simulink model "Furnace"  (R2020a)
settings: Solver=ode15s  StartTime=0  StopTime=27000  FixedStep=0.1  MaxStep=20  MinStep=1e-13  RelTol=1e-08  AbsTol=1e-09
undefined symbols (not defined in the file): agnostic_lqe_params, cont_reg, disturbance_type, F_aI_pid, F_aII_pid, input_type, k, lqe_params, LQR_params, LQRAgnostic_params, MPC_type, MPCDiscrete_function_parameters, MPCDiscreteAgnostic_function_parameters, MPCDiscreteDiffIntegralAgnostic_function_parameters, original_LQR_params, output_type, reg, single_butter_ss
libraries: simulink x35, cstblocks x10, mpclib x3
(part 3 of 8)

== system Furnace/Plant2/Turbine ==
  T_SH : Inport
  F_SH : Inport  Port=2
  p_drum : Inport  Port=3
  Scope : Scope
  Sum : Sum
  Transport Delay1 : TransportDelay  DelayTime=3  BufferSize=2048
  Transport Delay2 : TransportDelay  DelayTime=3  BufferSize=2048
  Turbine : MATLAB Function  TreatAsAtomicUnit=on
  W_net : Scope
  eta_TURB : Constant  Value=k.eta_TURB
  p_HP : Constant  Value=k.p_HP
  p_LP : Constant  Value=k.p_LP
  F_turb : Outport  VectorParamsAs1DForOutWhenUnconnected=off
  wires:
  T_SH/1 -> Turbine/1(T_SH)
  Turbine/1(W_el) -> Transport Delay1/1
  p_drum/1 -> Turbine/3(p_drum)
  F_SH/1 -> Transport Delay2/1, Turbine/2(F_SH)
  p_LP/1 -> Turbine/5(p_LP)
  Transport Delay1/1 -> Sum/1
  Transport Delay2/1 -> F_turb/1
  p_HP/1 -> Turbine/4(p_HP)
  Turbine/2(Q_turb) -> Scope/1
  eta_TURB/1 -> Turbine/6(eta_TURB)
  [W_fan] -> Sum/2
  Sum/1 -> W_net/1

== system Furnace/Actuator dynamics/Secondary air/Flue gas fan ==
  note: rpm of impeller
  note: Shaft torque
  PID signal : Inport
  Alpha : Gain  Gain=k.alpha_est_aII.*100
  Constant : Constant  Value=k.omega_T_aII
  Divide : Product  Inputs=*/
  Efficiency : Gain  Gain=k.mu_eff
  Gain : Gain  Gain=1/(k.I_aII)
  Gain4 : Gain  Gain=60/(2*pi)
  Integrator : Integrator  InitialCondition=reg.F_aII_fan_model_int
  "Linear mapping from rpm to volume flow " : Gain  Gain=k.map_aII
  "Maksimum power " : Gain  Gain=k.Pmax_aII
  Plus2 : Sum  Inputs=+-
  Square : Math  Operator=square  SignedPower=on  SaturateOnIntegerOverflow=on
  Square1 : Math  Operator=square  SignedPower=on  SaturateOnIntegerOverflow=on
  Static pressure converter : Gain  Gain=k.alpha_est_aII*2*3.1415/k.map_aII
  Switch : Switch  Criteria=u2 > Threshold  Threshold=k.omega_T_aII
  Volume flow : Outport  VectorParamsAs1DForOutWhenUnconnected=off
  Pressure difference : Outport  Port=2  VectorParamsAs1DForOutWhenUnconnected=off
  Power consumption : Outport  Port=3  VectorParamsAs1DForOutWhenUnconnected=off
  wires:
  Integrator/1 -> Square/1, Gain4/1, Switch/2, Switch/1, Square1/1
  Divide/1 -> Plus2/1
  Gain4/1 -> "Linear mapping from rpm to volume flow "/1
  Square/1 -> Static pressure converter/1
  Efficiency/1 -> Pressure difference/1
  "Maksimum power "/1 -> Power consumption/1, Divide/1
  Static pressure converter/1 -> Efficiency/1
  Alpha/1 -> Plus2/2
  Square1/1 -> Alpha/1
  Gain/1 -> Integrator/1
  Plus2/1 -> Gain/1
  PID signal/1 -> "Maksimum power "/1
  "Linear mapping from rpm to volume flow "/1 -> Volume flow/1
  Switch/1 -> Divide/2
  Constant/1 -> Switch/3

== system Furnace/Actuator dynamics/Waste and Primary air/Flue gas fan ==
  note: rpm of impeller
  note: Shaft torque
  PID signal : Inport
  Alpha : Gain  Gain=k.alpha_est_aII.*100
  Constant : Constant  Value=k.omega_T_aII
  Divide : Product  Inputs=*/
  Efficiency : Gain  Gain=k.mu_eff
  Gain : Gain  Gain=1/(k.I_aII)
  Gain4 : Gain  Gain=60/(2*pi)
  Integrator : Integrator  InitialCondition=reg.F_aI_fan_model_int
  "Linear mapping from rpm to volume flow " : Gain  Gain=k.map_aII
  "Maksimum power " : Gain  Gain=k.Pmax_aII
  Plus2 : Sum  Inputs=+-
  Square : Math  Operator=square  SignedPower=on  SaturateOnIntegerOverflow=on
  Square1 : Math  Operator=square  SignedPower=on  SaturateOnIntegerOverflow=on
  Static pressure converter : Gain  Gain=k.alpha_est_aII*2*3.1415/k.map_aII
  Switch : Switch  Criteria=u2 > Threshold  Threshold=k.omega_T_aII
  Volume flow : Outport  VectorParamsAs1DForOutWhenUnconnected=off
  Pressure difference : Outport  Port=2  VectorParamsAs1DForOutWhenUnconnected=off
  Power consumption : Outport  Port=3  VectorParamsAs1DForOutWhenUnconnected=off
  wires:
  Integrator/1 -> Square/1, Gain4/1, Switch/2, Switch/1, Square1/1
  Divide/1 -> Plus2/1
  Gain4/1 -> "Linear mapping from rpm to volume flow "/1
  Square/1 -> Static pressure converter/1
  Efficiency/1 -> Pressure difference/1
  "Maksimum power "/1 -> Power consumption/1, Divide/1
  Static pressure converter/1 -> Efficiency/1
  Alpha/1 -> Plus2/2
  Square1/1 -> Alpha/1
  Gain/1 -> Integrator/1
  Plus2/1 -> Gain/1
  PID signal/1 -> "Maksimum power "/1
  "Linear mapping from rpm to volume flow "/1 -> Volume flow/1
  Switch/1 -> Divide/2
  Constant/1 -> Switch/3

== system Furnace/Controller/MPC_subsystem/LQG_controller ==
  noisy_y : Inport  OutDataTypeStr=double
  v in : Inport  Port=2
  u in : Inport  Port=3
  Controler_reference : Inport  Port=4  OutDataTypeStr=double
  Controller_battery : Subsystem
  Enforce proper size : Selector  InputPortWidth=original_LQR_params.N_refs  IndexOptions=Index vector (dialog)  Indices=1:original_LQR_params.N_refs  OutputSizes=1
  Extended x1 : Concatenate  NumInputs=3
  Extended x2 : Concatenate  NumInputs=3
  Ground : Ground
  Ground1 : Ground
  Kalman filter battery : Subsystem
      settings: PortSchema="{\"entries\":[{\"content\":{\"sides\":[{\"content\":{\"connectorIds\":[\"In1\",\"In2\",\"In3\"]},\"type\":\"ConnectorPlacement.EquallySpacedRectSide\",\"uuid\":\"1c993a74-2ebc-4ff1-8a36-810b6615b91b\"},{\"content\":{\"connectorIds\":[\"Out1\",\"Out2\",\"Out3\",\"Out4\"],\"side\":\"RIGHT\"},\"type\":\"ConnectorPlacement.EquallySpacedRectSide\",\"uuid\":\"f47ce850-e8b0-4437-a8da-01c6ea316d70\"},{\"content\":{\"connectorIds\":[],\"side\":\"TOP\"},\"type\":\"ConnectorPlacement.EquallySpacedRectSide\",\"uuid\":\"49075f58-3726-424f-842a-93e04b24d953\"},{\"content\":{\"connectorIds\":[\"In4\"],\"side\":\"BOTTOM\"},\"type\":\"ConnectorPlacement.EquallySpacedRectSide\",\"uuid\":\"0a8cab2c-6cc5-4573-a1bf-983f74a1ee29\"}]},\"type\":\"ConnectorPlacement.EquallySpacedConnector\",\"uuid\":\"113553bc-ba05-4a25-98d3-042b5b48218e\"}],\"packageUris\":[\"http://schema.mathworks.com/mf0/Connector/19700101\"],\"version\":\"1.0\"}"
  Manual Switch : ManualSwitch
  Manual Switch1 : ManualSwitch
  Scope : Scope
  Selector4 : Selector  InputPortWidth=4  IndexOptions=Index vector (dialog)  Indices=1:4  OutputSizes=1
  Selector5 : Selector  InputPortWidth=4  IndexOptions=Index vector (dialog)  Indices=1:4  OutputSizes=1
  u_mpc : Outport
  y_hat : Outport  Port=2
  wires:
  Controler_reference/1 -> Enforce proper size/1
  u in/1 -> Selector4/1
  Enforce proper size/1 -> Controller_battery/4(ref), Kalman filter battery/4(ref)
  Kalman filter battery/2(Integrated_measurement_errors) -> Extended x2/3, Extended x1/3, Scope/1
  noisy_y/1 -> Kalman filter battery/3(y)
  Kalman filter battery/1(y_MPC_hat) -> y_hat/1
  Selector5/1 -> u_mpc/1
  Selector4/1 -> Extended x1/2, Extended x2/2, Controller_battery/2(u_used), Kalman filter battery/1(u_in)
  Controller_battery/1(v_grate) -> Selector5/1
  v in/1 -> Kalman filter battery/2(v in)
  Kalman filter battery/4(x_hat_agnostic) -> Extended x2/1
  Manual Switch/1 -> Controller_battery/1(x_lqe)
  Manual Switch1/1 -> Controller_battery/3(x_lqe_agnostic)
  Kalman filter battery/3(x_hat_assuming) -> Extended x1/1
  Extended x1/1 -> Manual Switch/1
  Extended x2/1 -> Manual Switch1/1
  Ground/1 -> Manual Switch/2
  Ground1/1 -> Manual Switch1/2

== system Furnace/Controller/Subsystem/Butterworth_filter1 ==
  In : Inport
  Gain2 : Gain  Gain=single_butter_ss.B  Multiplication=Matrix(K*u)
  Gain3 : Gain  Gain=single_butter_ss.C  Multiplication=Matrix(K*u)
  Gain4 : Gain  Gain=single_butter_ss.A  Multiplication=Matrix(K*u)
  Integrator : Integrator
  Sum : Sum  Inputs=|++
  Filtered : Outport
  wires:
  Gain3/1 -> Filtered/1
  In/1 -> Gain2/1
  Gain2/1 -> Sum/1
  Integrator/1 -> Gain4/1, Gain3/1
  Gain4/1 -> Sum/2
  Sum/1 -> Integrator/1

== system Furnace/Controller/Subsystem/Butterworth_filter2 ==
  In : Inport
  Gain2 : Gain  Gain=single_butter_ss.B  Multiplication=Matrix(K*u)
  Gain3 : Gain  Gain=single_butter_ss.C  Multiplication=Matrix(K*u)
  Gain4 : Gain  Gain=single_butter_ss.A  Multiplication=Matrix(K*u)
  Integrator : Integrator
  Sum : Sum  Inputs=|++
  Filtered : Outport
  wires:
  Sum/1 -> Integrator/1
  Gain4/1 -> Sum/2
  Integrator/1 -> Gain3/1, Gain4/1
  Gain2/1 -> Sum/1
  In/1 -> Gain2/1
  Gain3/1 -> Filtered/1

== system Furnace/Controller/Subsystem/Butterworth_filter3 ==
  In : Inport
  Gain2 : Gain  Gain=single_butter_ss.B  Multiplication=Matrix(K*u)
  Gain3 : Gain  Gain=single_butter_ss.C  Multiplication=Matrix(K*u)
  Gain4 : Gain  Gain=single_butter_ss.A  Multiplication=Matrix(K*u)
  Integrator : Integrator
  Sum : Sum  Inputs=|++
  Filtered : Outport
  wires:
  Gain3/1 -> Filtered/1
  In/1 -> Gain2/1
  Gain2/1 -> Sum/1
  Integrator/1 -> Gain4/1, Gain3/1
  Gain4/1 -> Sum/2
  Sum/1 -> Integrator/1

== system Furnace/Deprecated, slow loop/Actuator dynamics/Grate speed ==
  v_grate_reg_in : Inport
  v_grate_out : Outport  VectorParamsAs1DForOutWhenUnconnected=off
  wires:
  v_grate_reg_in/1 -> v_grate_out/1  "v_grate"

== system Furnace/Deprecated, slow loop/Actuator dynamics/Secondary air ==
  F_aII_reg_in : Inport
  Flue gas fan : Subsystem
  PID Controller : simulink/Continuous/PID Controller  Controller=PI  Form=Parallel  TimeDomain=Continuous-time  UseExternalTs=off  SampleTime=1  IntegratorMethod=Forward Euler  FilterMethod=Forward Euler  ControllerParametersSource=internal  P=reg.Kp_fan  I=reg.Ki_fan  D=0  UseFilter=on  N=100  TunerSelectOption=Transfer Function Based (PID Tuner App)  InitialConditionSource=internal  InitialConditionForIntegrator=reg.F_aII_fan_PID_int  InitialConditionForFilter=0  DifferentiatorICPrevScaledInput=0  ExternalReset=none  TrackingMode=off  Kt=1  LimitOutput=off  UpperSaturationLimit=inf  LowerSaturationLimit=-inf  LinearizeAsGain=on  AntiWindupMode=none  Kb=1  POutMin=[]  POutMax=[]  IOutMin=[]  IOutMax=[]  DOutMin=[]  DOutMax=[]  NOutMin=[]  NOutMax=[]  SumOutMin=[]  SumOutMax=[]  SaturationOutMin=[]  SaturationOutMax=[]  PParamMin=[]  PParamMax=[]  IParamMin=[]  IParamMax=[]  DParamMin=[]  DParamMax=[]  NParamMin=[]  NParamMax=[]  KbParamMin=[]  KbParamMax=[]  KtParamMin=[]  KtParamMax=[]  KbOutMin=[]  KbOutMax=[]  KtOutMin=[]  KtOutMax=[]  IntegratorOutMin=[]  IntegratorOutMax=[]  FilterOutMin=[]  FilterOutMax=[]  SumI1OutMin=[]  SumI1OutMax=[]  SumI2OutMin=[]  SumI2OutMax=[]  SumI3OutMin=[]  SumI3OutMax=[]  SumI4OutMin=[]  SumI4OutMax=[]  SumDOutMin=[]  SumDOutMax=[]  DifferentiatorOutMin=[]  DifferentiatorOutMax=[]  FilterDiffOutCoefMin=[]  FilterDiffOutCoefMax=[]  ReciprocalOutMin=[]  ReciprocalOutMax=[]  SumDenOutMin=[]  SumDenOutMax=[]  SumNumOutMin=[]  SumNumOutMax=[]  DivideOutMin=[]  DivideOutMax=[]  UdiffTsProdOutMin=[]  UdiffTsProdOutMax=[]  NTsProdOutMin=[]  NTsProdOutMax=[]  UintegralTsProdOutMin=[]  UintegralTsProdOutMax=[]  UngainTsProdOutMin=[]  UngainTsProdOutMax=[]  IntegratorContinuousStateAttributes=''  IntegratorStateMustResolveToSignalObject=off  IntegratorRTWStateStorageClass=Auto  FilterContinuousStateAttributes=''  FilterStateMustResolveToSignalObject=off  FilterRTWStateStorageClass=Auto  ParallelPVariant=InternalParameters  IdealPVariant=Disabled  IVariant=InternalParameters  DVariant=Disabled  IntegratorVariant=Continuous  SatVariant=Disabled  AWVariant=Passthrough  PCopyVariant=Disabled  TRVariant=Disabled  FdbkBlocksVariant=Forward  IdealPFdbkVariant=Disabled  SatFdbkVariant=Disabled  DerivativeFilterVariant=Disabled  NVariant=Disabled  NCopyVariant=Disabled_SignalSpec  FilterICVariant=Disabled  IntegratorICVariant=InternalICs  ExternalResetVariant=Disabled  TRSumVariant=Passthrough  SumFdbkVariant=Disabled  SumVariant=Sum_PI  TsampFilterVariant=InternalTs  TsampNgainVariant=Passthrough  TsampIntegralVariant=Passthrough
  Sum1 : Sum  Inputs=|+-
  F_aII_out : Outport  VectorParamsAs1DForOutWhenUnconnected=off
  wires:
  Sum1/1 -> PID Controller/1
  PID Controller/1 -> Flue gas fan/1(PID signal)
  Flue gas fan/1(Volume flow) -> F_aII_out/1, Sum1/2
  F_aII_reg_in/1 -> Sum1/1

== system Furnace/Deprecated, slow loop/Actuator dynamics/Waste and Primary air ==
  "F_aI_reg_in " : Inport
  F_w_in_reg : Inport  Port=2
  Constant2 : Constant  Value=reg.const_F_aI_dist
  Fiw_in1 : Constant  Value=k.w_w_in
  Flue gas fan : Subsystem
  "For now(Bad hack) " : Gain  Gain=1./(reg.const_F_aI_dist* length(reg.const_F_aI_dist))
  PID Controller : simulink/Continuous/PID Controller  Controller=PI  Form=Parallel  TimeDomain=Continuous-time  UseExternalTs=off  SampleTime=1  IntegratorMethod=Forward Euler  FilterMethod=Forward Euler  ControllerParametersSource=internal  P=reg.Kp_fan  I=reg.Ki_fan  D=0  UseFilter=on  N=100  TunerSelectOption=Transfer Function Based (PID Tuner App)  InitialConditionSource=internal  InitialConditionForIntegrator=reg.F_aI_fan_PID_int  InitialConditionForFilter=0  DifferentiatorICPrevScaledInput=0  ExternalReset=none  TrackingMode=off  Kt=1  LimitOutput=off  UpperSaturationLimit=inf  LowerSaturationLimit=-inf  LinearizeAsGain=on  AntiWindupMode=none  Kb=1  POutMin=[]  POutMax=[]  IOutMin=[]  IOutMax=[]  DOutMin=[]  DOutMax=[]  NOutMin=[]  NOutMax=[]  SumOutMin=[]  SumOutMax=[]  SaturationOutMin=[]  SaturationOutMax=[]  PParamMin=[]  PParamMax=[]  IParamMin=[]  IParamMax=[]  DParamMin=[]  DParamMax=[]  NParamMin=[]  NParamMax=[]  KbParamMin=[]  KbParamMax=[]  KtParamMin=[]  KtParamMax=[]  KbOutMin=[]  KbOutMax=[]  KtOutMin=[]  KtOutMax=[]  IntegratorOutMin=[]  IntegratorOutMax=[]  FilterOutMin=[]  FilterOutMax=[]  SumI1OutMin=[]  SumI1OutMax=[]  SumI2OutMin=[]  SumI2OutMax=[]  SumI3OutMin=[]  SumI3OutMax=[]  SumI4OutMin=[]  SumI4OutMax=[]  SumDOutMin=[]  SumDOutMax=[]  DifferentiatorOutMin=[]  DifferentiatorOutMax=[]  FilterDiffOutCoefMin=[]  FilterDiffOutCoefMax=[]  ReciprocalOutMin=[]  ReciprocalOutMax=[]  SumDenOutMin=[]  SumDenOutMax=[]  SumNumOutMin=[]  SumNumOutMax=[]  DivideOutMin=[]  DivideOutMax=[]  UdiffTsProdOutMin=[]  UdiffTsProdOutMax=[]  NTsProdOutMin=[]  NTsProdOutMax=[]  UintegralTsProdOutMin=[]  UintegralTsProdOutMax=[]  UngainTsProdOutMin=[]  UngainTsProdOutMax=[]  IntegratorContinuousStateAttributes=''  IntegratorStateMustResolveToSignalObject=off  IntegratorRTWStateStorageClass=Auto  FilterContinuousStateAttributes=''  FilterStateMustResolveToSignalObject=off  FilterRTWStateStorageClass=Auto  ParallelPVariant=InternalParameters  IdealPVariant=Disabled  IVariant=InternalParameters  DVariant=Disabled  IntegratorVariant=Continuous  SatVariant=Disabled  AWVariant=Passthrough  PCopyVariant=Disabled  TRVariant=Disabled  FdbkBlocksVariant=Forward  IdealPFdbkVariant=Disabled  SatFdbkVariant=Disabled  DerivativeFilterVariant=Disabled  NVariant=Disabled  NCopyVariant=Disabled_SignalSpec  FilterICVariant=Disabled  IntegratorICVariant=InternalICs  ExternalResetVariant=Disabled  TRSumVariant=Passthrough  SumFdbkVariant=Disabled  SumVariant=Sum_PI  TsampFilterVariant=InternalTs  TsampNgainVariant=Passthrough  TsampIntegralVariant=Passthrough
  Product : Product
  Product1 : Product
  Square perturbation : SignalGenerator  WaveForm=square  Amplitude=reg.F_w_pert_amp  Frequency=reg.F_w_pert_freq
  Sum : Sum  Inputs=++|
  Sum of Elements : Sum  Inputs=+
  Sum1 : Sum  Inputs=|+-
  Sum2 : Sum  Inputs=+
  Fi_w_out : Outport  VectorParamsAs1DForOutWhenUnconnected=off
  Fi_aI_out : Outport  Port=2  VectorParamsAs1DForOutWhenUnconnected=off
  wires:
  Fiw_in1/1 -> Product/2
  Product/1 -> Fi_w_out/1
  Product1/1 -> Fi_aI_out/1, Sum of Elements/1  "F_aI_out"
  F_w_in_reg/1 -> Sum/2  "F_w_in"
  Sum/1 -> Product/1
  Square perturbation/1 -> Sum/1
  PID Controller/1 -> Flue gas fan/1(PID signal)
  Sum1/1 -> PID Controller/1
  Constant2/1 -> Product1/2
  Flue gas fan/1(Volume flow) -> Sum1/2, Product1/1
  "For now(Bad hack) "/1 -> Sum2/1
  "F_aI_reg_in "/1 -> "For now(Bad hack) "/1  "F_aI_out"
  Sum2/1 -> Sum1/1

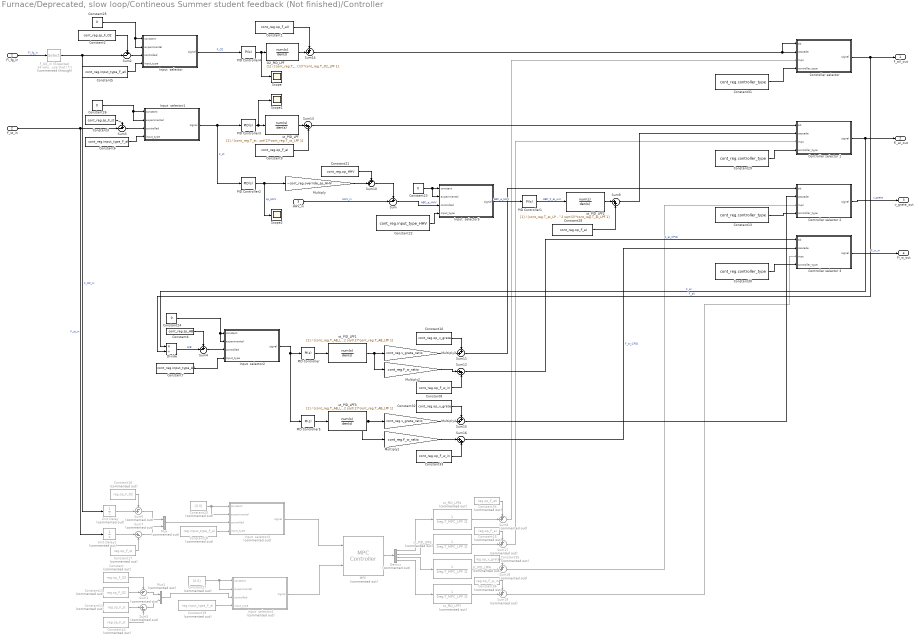
== system Furnace/Deprecated, slow loop/Contineous Summer student feedback (Not finished)/Controller ==
  Fi_fg_in : Inport
  F_st_in : Inport  Port=2
  HHV_in : Inport  Port=3
  Constant : Constant  Commented=on  Value=reg.op_F_O2
  Constant1 : Constant  Value=cont_reg.op_F_aII
  Constant10 : Constant  Value=cont_reg.op_v_grate
  Constant11 : Constant  Commented=on  Value=reg.sp_F_st
  Constant12 : Constant  Commented=on  Value=reg.sp_F_O2
  Constant{13,29..31} (4 alike) : Constant  Value=cont_reg.controller_type
  Constant14 : Constant  Commented=on  Value=reg.op_F_st
  Constant15 : Constant  Commented=on  Value=reg.op_F_aI
  Constant16 : Constant  Commented=on  Value=reg.op_F_O2
  Constant17 : Constant  Commented=on  Value=reg.op_F_st
  Constant18 : Constant  Commented=on  Value=reg.input_type_F_aI
  Constant19 : Constant  Commented=on  Value=reg.input_type_F_aI
  Constant2 : Constant  Value=cont_reg.sp_F_O2
  Constant20 : Constant  Commented=on  Value=[0 0]
  Constant21 : Constant  Value=cont_reg.op_HHV
  Constant22 : Constant  Value=cont_reg.input_type_HHV
  Constant{23..26} (4 alike) : Constant  Value=0
  Constant27 : Constant  Commented=on  Value=[0 0]
  Constant28 : Constant  Value=cont_reg.op_F_aI
  Constant3 : Constant  Value=cont_reg.sp_F_st
  Constant32 : Constant  Value=cont_reg.op_v_grate
  Constant33 : Constant  Value=cont_reg.op_F_w_in
  Constant34 : Constant  Commented=on  Value=reg.op_F_aII
  Constant35 : Constant  Commented=on  Value=reg.op_v_grate
  Constant36 : Constant  Commented=on  Value=reg.op_F_w_in
  Constant4 : Constant  Value=cont_reg.sp_AB
  Constant5 : Constant  Value=cont_reg.input_type_F_aII
  Constant6 : Constant  Value=cont_reg.input_type_F_aI
  Constant7 : Constant  Value=cont_reg.input_type_AB
  Constant8 : Constant  Value=cont_reg.op_F_w_in
  Constant9 : Constant  Value=cont_reg.op_F_aI
  "Controller selector " : MATLAB Function  TreatAsAtomicUnit=on
  Controller selector 1 : MATLAB Function  TreatAsAtomicUnit=on
  Controller selector 2 : MATLAB Function  TreatAsAtomicUnit=on
  Controller selector 3 : MATLAB Function  TreatAsAtomicUnit=on
  Demux : Demux  Commented=on
  Divide : Product  Inputs=*/  OutMin=[-100]  OutMax=[100]
  "F_O2_in (Expected 14 values, new simulator does not use that (?))" : Selector  Commented=through  InputPortWidth=12  IndexOptions=Index vector (dialog)  Indices=[4]  OutputSizes=1
  Input  selector : MATLAB Function  TreatAsAtomicUnit=on
  Input  selector1 : MATLAB Function  TreatAsAtomicUnit=on
  Input  selector2 : MATLAB Function  TreatAsAtomicUnit=on
  Input  selector3 : MATLAB Function  Commented=on  TreatAsAtomicUnit=on
  Input  selector4 : MATLAB Function  Commented=on  TreatAsAtomicUnit=on
  Input  selector5 : MATLAB Function  TreatAsAtomicUnit=on
  MPC : mpclib/MPC Controller  Commented=on  SCDEnableBlockLinearizationSpecification=on  mpcobj=lmpc  is_multiple=0  enable_value=0  return_u0=off  updateMPCinCallerWorkspace=on  md_inport=off  mv_inport=off  uref_inport=off  return_cost=off  return_mvseq=off  return_qpstatus=off  return_xseq=off  return_state=off  return_ovseq=off  state_inport=off  umin_inport=off  umax_inport=off  ymin_inport=off  ymax_inport=off  cc_inport=off  ywt_inport=off  uwt_inport=off  duwt_inport=off  rhoeps_inport=off  pm_inport=off  MaximumP=10  HorizonChoice=FixedHorizon  n_ts=20  n_p=50  n_mv=4  n_md=0  n_ud=0  n_mo=2  n_uo=0  BlockDataType=double  SampleTimeInherited=off  switch_inport=off
  Multiply : Gain  Gain=~cont_reg.override_sp_HHV
  Multiply1 : Gain  Gain=cont_reg.F_w_ratio
  Multiply2 : Gain  Gain=cont_reg.F_w_ratio
  Multiply3 : Gain  Gain=cont_reg.v_grate_ratio
  Multiply4 : Gain  Gain=cont_reg.v_grate_ratio
  Mux : Mux  Commented=on  Inputs=2
  Mux1 : Mux  Commented=on  Inputs=2
  O2_PID_LPF : TransferFcn  Denominator=[cont_reg.T_O2_LPF^2 sqrt(2)*cont_reg.T_O2_LPF 1]
  PID Controller : simulink/Continuous/PID Controller  Controller=PI  Form=Parallel  TimeDomain=Continuous-time  UseExternalTs=off  SampleTime=1  IntegratorMethod=Forward Euler  FilterMethod=Forward Euler  ControllerParametersSource=internal  P=cont_reg.Kp_AB  I=cont_reg.Ki_AB  D=0  UseFilter=on  N=100  TunerSelectOption=Transfer Function Based (PID Tuner App)  InitialConditionSource=internal  InitialConditionForIntegrator=0  InitialConditionForFilter=0  DifferentiatorICPrevScaledInput=0  ExternalReset=none  TrackingMode=off  Kt=1  LimitOutput=off  UpperSaturationLimit=inf  LowerSaturationLimit=-inf  LinearizeAsGain=on  AntiWindupMode=none  Kb=1  POutMin=[]  POutMax=[]  IOutMin=[]  IOutMax=[]  DOutMin=[]  DOutMax=[]  NOutMin=[]  NOutMax=[]  SumOutMin=[]  SumOutMax=[]  SaturationOutMin=[]  SaturationOutMax=[]  PParamMin=[]  PParamMax=[]  IParamMin=[]  IParamMax=[]  DParamMin=[]  DParamMax=[]  NParamMin=[]  NParamMax=[]  KbParamMin=[]  KbParamMax=[]  KtParamMin=[]  KtParamMax=[]  KbOutMin=[]  KbOutMax=[]  KtOutMin=[]  KtOutMax=[]  IntegratorOutMin=[]  IntegratorOutMax=[]  FilterOutMin=[]  FilterOutMax=[]  SumI1OutMin=[]  SumI1OutMax=[]  SumI2OutMin=[]  SumI2OutMax=[]  SumI3OutMin=[]  SumI3OutMax=[]  SumI4OutMin=[]  SumI4OutMax=[]  SumDOutMin=[]  SumDOutMax=[]  DifferentiatorOutMin=[]  DifferentiatorOutMax=[]  FilterDiffOutCoefMin=[]  FilterDiffOutCoefMax=[]  ReciprocalOutMin=[]  ReciprocalOutMax=[]  SumDenOutMin=[]  SumDenOutMax=[]  SumNumOutMin=[]  SumNumOutMax=[]  DivideOutMin=[]  DivideOutMax=[]  UdiffTsProdOutMin=[]  UdiffTsProdOutMax=[]  NTsProdOutMin=[]  NTsProdOutMax=[]  UintegralTsProdOutMin=[]  UintegralTsProdOutMax=[]  UngainTsProdOutMin=[]  UngainTsProdOutMax=[]  IntegratorContinuousStateAttributes=''  IntegratorStateMustResolveToSignalObject=off  IntegratorRTWStateStorageClass=Auto  FilterContinuousStateAttributes=''  FilterStateMustResolveToSignalObject=off  FilterRTWStateStorageClass=Auto  ParallelPVariant=InternalParameters  IdealPVariant=Disabled  IVariant=InternalParameters  DVariant=Disabled  IntegratorVariant=Continuous  SatVariant=Disabled  AWVariant=Passthrough  PCopyVariant=Disabled  TRVariant=Disabled  FdbkBlocksVariant=Forward  IdealPFdbkVariant=Disabled  SatFdbkVariant=Disabled  DerivativeFilterVariant=Disabled  NVariant=Disabled  NCopyVariant=Disabled_SignalSpec  FilterICVariant=Disabled  IntegratorICVariant=InternalICs  ExternalResetVariant=Disabled  TRSumVariant=Passthrough  SumFdbkVariant=Disabled  SumVariant=Sum_PI  TsampFilterVariant=InternalTs  TsampNgainVariant=Passthrough  TsampIntegralVariant=Passthrough
  PID Controller1 : simulink/Continuous/PID Controller  Controller=PI  Form=Parallel  TimeDomain=Continuous-time  UseExternalTs=off  SampleTime=1  IntegratorMethod=Forward Euler  FilterMethod=Forward Euler  ControllerParametersSource=internal  P=cont_reg.Kp_HHV  I=cont_reg.Ki_HHV  D=0  UseFilter=on  N=100  TunerSelectOption=Transfer Function Based (PID Tuner App)  InitialConditionSource=internal  InitialConditionForIntegrator=0  InitialConditionForFilter=0  DifferentiatorICPrevScaledInput=0  ExternalReset=none  TrackingMode=off  Kt=1  LimitOutput=off  UpperSaturationLimit=inf  LowerSaturationLimit=-inf  LinearizeAsGain=on  AntiWindupMode=none  Kb=1  POutMin=[]  POutMax=[]  IOutMin=[]  IOutMax=[]  DOutMin=[]  DOutMax=[]  NOutMin=[]  NOutMax=[]  SumOutMin=[]  SumOutMax=[]  SaturationOutMin=[]  SaturationOutMax=[]  PParamMin=[]  PParamMax=[]  IParamMin=[]  IParamMax=[]  DParamMin=[]  DParamMax=[]  NParamMin=[]  NParamMax=[]  KbParamMin=[]  KbParamMax=[]  KtParamMin=[]  KtParamMax=[]  KbOutMin=[]  KbOutMax=[]  KtOutMin=[]  KtOutMax=[]  IntegratorOutMin=[]  IntegratorOutMax=[]  FilterOutMin=[]  FilterOutMax=[]  SumI1OutMin=[]  SumI1OutMax=[]  SumI2OutMin=[]  SumI2OutMax=[]  SumI3OutMin=[]  SumI3OutMax=[]  SumI4OutMin=[]  SumI4OutMax=[]  SumDOutMin=[]  SumDOutMax=[]  DifferentiatorOutMin=[]  DifferentiatorOutMax=[]  FilterDiffOutCoefMin=[]  FilterDiffOutCoefMax=[]  ReciprocalOutMin=[]  ReciprocalOutMax=[]  SumDenOutMin=[]  SumDenOutMax=[]  SumNumOutMin=[]  SumNumOutMax=[]  DivideOutMin=[]  DivideOutMax=[]  UdiffTsProdOutMin=[]  UdiffTsProdOutMax=[]  NTsProdOutMin=[]  NTsProdOutMax=[]  UintegralTsProdOutMin=[]  UintegralTsProdOutMax=[]  UngainTsProdOutMin=[]  UngainTsProdOutMax=[]  IntegratorContinuousStateAttributes=''  IntegratorStateMustResolveToSignalObject=off  IntegratorRTWStateStorageClass=Auto  FilterContinuousStateAttributes=''  FilterStateMustResolveToSignalObject=off  FilterRTWStateStorageClass=Auto  ParallelPVariant=InternalParameters  IdealPVariant=Disabled  IVariant=InternalParameters  DVariant=Disabled  IntegratorVariant=Continuous  SatVariant=Disabled  AWVariant=Passthrough  PCopyVariant=Disabled  TRVariant=Disabled  FdbkBlocksVariant=Forward  IdealPFdbkVariant=Disabled  SatFdbkVariant=Disabled  DerivativeFilterVariant=Disabled  NVariant=Disabled  NCopyVariant=Disabled_SignalSpec  FilterICVariant=Disabled  IntegratorICVariant=InternalICs  ExternalResetVariant=Disabled  TRSumVariant=Passthrough  SumFdbkVariant=Disabled  SumVariant=Sum_PI  TsampFilterVariant=InternalTs  TsampNgainVariant=Passthrough  TsampIntegralVariant=Passthrough
  PID Controller2 : simulink/Continuous/PID Controller  Controller=PID  Form=Parallel  TimeDomain=Continuous-time  UseExternalTs=off  SampleTime=1  IntegratorMethod=Forward Euler  FilterMethod=Forward Euler  ControllerParametersSource=internal  P=cont_reg.Kp_st_HHV  I=cont_reg.Ki_st_HHV  D=cont_reg.Kd_st_HHV  UseFilter=on  N=100  TunerSelectOption=Transfer Function Based (PID Tuner App)  InitialConditionSource=internal  InitialConditionForIntegrator=0.001  InitialConditionForFilter=0  DifferentiatorICPrevScaledInput=0  ExternalReset=none  TrackingMode=off  Kt=1  LimitOutput=off  UpperSaturationLimit=inf  LowerSaturationLimit=1  LinearizeAsGain=on  AntiWindupMode=none  Kb=1  POutMin=[]  POutMax=[]  IOutMin=[]  IOutMax=[]  DOutMin=[]  DOutMax=[]  NOutMin=[]  NOutMax=[]  SumOutMin=[]  SumOutMax=[]  SaturationOutMin=[]  SaturationOutMax=[]  PParamMin=[]  PParamMax=[]  IParamMin=[]  IParamMax=[]  DParamMin=[]  DParamMax=[]  NParamMin=[]  NParamMax=[]  KbParamMin=[]  KbParamMax=[]  KtParamMin=[]  KtParamMax=[]  KbOutMin=[]  KbOutMax=[]  KtOutMin=[]  KtOutMax=[]  IntegratorOutMin=[]  IntegratorOutMax=[]  FilterOutMin=[]  FilterOutMax=[]  SumI1OutMin=[]  SumI1OutMax=[]  SumI2OutMin=[]  SumI2OutMax=[]  SumI3OutMin=[]  SumI3OutMax=[]  SumI4OutMin=[]  SumI4OutMax=[]  SumDOutMin=[]  SumDOutMax=[]  DifferentiatorOutMin=[]  DifferentiatorOutMax=[]  FilterDiffOutCoefMin=[]  FilterDiffOutCoefMax=[]  ReciprocalOutMin=[]  ReciprocalOutMax=[]  SumDenOutMin=[]  SumDenOutMax=[]  SumNumOutMin=[]  SumNumOutMax=[]  DivideOutMin=[]  DivideOutMax=[]  UdiffTsProdOutMin=[]  UdiffTsProdOutMax=[]  NTsProdOutMin=[]  NTsProdOutMax=[]  UintegralTsProdOutMin=[]  UintegralTsProdOutMax=[]  UngainTsProdOutMin=[]  UngainTsProdOutMax=[]  IntegratorContinuousStateAttributes='F_st'  IntegratorStateMustResolveToSignalObject=off  IntegratorRTWStateStorageClass=Auto  FilterContinuousStateAttributes=''  FilterStateMustResolveToSignalObject=off  FilterRTWStateStorageClass=Auto  ParallelPVariant=InternalParameters  IdealPVariant=Disabled  IVariant=InternalParameters  DVariant=InternalParameters  IntegratorVariant=Continuous  SatVariant=Disabled  AWVariant=Passthrough  PCopyVariant=Disabled  TRVariant=Disabled  FdbkBlocksVariant=Forward  IdealPFdbkVariant=Disabled  SatFdbkVariant=Disabled  DerivativeFilterVariant=ContFilter  NVariant=InternalParameters  NCopyVariant=Disabled  FilterICVariant=InternalICsFilter  IntegratorICVariant=InternalICs  ExternalResetVariant=Disabled  TRSumVariant=Passthrough  SumFdbkVariant=Disabled  SumVariant=Sum_PID  TsampFilterVariant=InternalTs  TsampNgainVariant=Passthrough  TsampIntegralVariant=Passthrough
  PID Controller3 : simulink/Continuous/PID Controller  Controller=PID  Form=Parallel  TimeDomain=Continuous-time  UseExternalTs=off  SampleTime=1  IntegratorMethod=Forward Euler  FilterMethod=Forward Euler  ControllerParametersSource=internal  P=cont_reg.Kp_st  I=cont_reg.Ki_st  D=cont_reg.Kd_st  UseFilter=on  N=100  TunerSelectOption=Transfer Function Based (PID Tuner App)  InitialConditionSource=internal  InitialConditionForIntegrator=0  InitialConditionForFilter=0  DifferentiatorICPrevScaledInput=0  ExternalReset=none  TrackingMode=off  Kt=1  LimitOutput=off  UpperSaturationLimit=inf  LowerSaturationLimit=1  LinearizeAsGain=on  AntiWindupMode=none  Kb=1  POutMin=[]  POutMax=[]  IOutMin=[]  IOutMax=[]  DOutMin=[]  DOutMax=[]  NOutMin=[]  NOutMax=[]  SumOutMin=[]  SumOutMax=[]  SaturationOutMin=[]  SaturationOutMax=[]  PParamMin=[]  PParamMax=[]  IParamMin=[]  IParamMax=[]  DParamMin=[]  DParamMax=[]  NParamMin=[]  NParamMax=[]  KbParamMin=[]  KbParamMax=[]  KtParamMin=[]  KtParamMax=[]  KbOutMin=[]  KbOutMax=[]  KtOutMin=[]  KtOutMax=[]  IntegratorOutMin=[]  IntegratorOutMax=[]  FilterOutMin=[]  FilterOutMax=[]  SumI1OutMin=[]  SumI1OutMax=[]  SumI2OutMin=[]  SumI2OutMax=[]  SumI3OutMin=[]  SumI3OutMax=[]  SumI4OutMin=[]  SumI4OutMax=[]  SumDOutMin=[]  SumDOutMax=[]  DifferentiatorOutMin=[]  DifferentiatorOutMax=[]  FilterDiffOutCoefMin=[]  FilterDiffOutCoefMax=[]  ReciprocalOutMin=[]  ReciprocalOutMax=[]  SumDenOutMin=[]  SumDenOutMax=[]  SumNumOutMin=[]  SumNumOutMax=[]  DivideOutMin=[]  DivideOutMax=[]  UdiffTsProdOutMin=[]  UdiffTsProdOutMax=[]  NTsProdOutMin=[]  NTsProdOutMax=[]  UintegralTsProdOutMin=[]  UintegralTsProdOutMax=[]  UngainTsProdOutMin=[]  UngainTsProdOutMax=[]  IntegratorContinuousStateAttributes='F_st'  IntegratorStateMustResolveToSignalObject=off  IntegratorRTWStateStorageClass=Auto  FilterContinuousStateAttributes=''  FilterStateMustResolveToSignalObject=off  FilterRTWStateStorageClass=Auto  ParallelPVariant=InternalParameters  IdealPVariant=Disabled  IVariant=InternalParameters  DVariant=InternalParameters  IntegratorVariant=Continuous  SatVariant=Disabled  AWVariant=Passthrough  PCopyVariant=Disabled  TRVariant=Disabled  FdbkBlocksVariant=Forward  IdealPFdbkVariant=Disabled  SatFdbkVariant=Disabled  DerivativeFilterVariant=ContFilter  NVariant=InternalParameters  NCopyVariant=Disabled  FilterICVariant=InternalICsFilter  IntegratorICVariant=InternalICs  ExternalResetVariant=Disabled  TRSumVariant=Passthrough  SumFdbkVariant=Disabled  SumVariant=Sum_PID  TsampFilterVariant=InternalTs  TsampNgainVariant=Passthrough  TsampIntegralVariant=Passthrough
  PID Controller4 : simulink/Continuous/PID Controller  Controller=PI  Form=Parallel  TimeDomain=Continuous-time  UseExternalTs=off  SampleTime=1  IntegratorMethod=Forward Euler  FilterMethod=Forward Euler  ControllerParametersSource=internal  P=cont_reg.Kp_O2  I=cont_reg.Ki_O2  D=0  UseFilter=on  N=100  TunerSelectOption=Transfer Function Based (PID Tuner App)  InitialConditionSource=internal  InitialConditionForIntegrator=0.001  InitialConditionForFilter=0  DifferentiatorICPrevScaledInput=0  ExternalReset=none  TrackingMode=off  Kt=1  LimitOutput=off  UpperSaturationLimit=inf  LowerSaturationLimit=1  LinearizeAsGain=on  AntiWindupMode=none  Kb=1  POutMin=[]  POutMax=[]  IOutMin=[]  IOutMax=[]  DOutMin=[]  DOutMax=[]  NOutMin=[]  NOutMax=[]  SumOutMin=[]  SumOutMax=[]  SaturationOutMin=[]  SaturationOutMax=[]  PParamMin=[]  PParamMax=[]  IParamMin=[]  IParamMax=[]  DParamMin=[]  DParamMax=[]  NParamMin=[]  NParamMax=[]  KbParamMin=[]  KbParamMax=[]  KtParamMin=[]  KtParamMax=[]  KbOutMin=[]  KbOutMax=[]  KtOutMin=[]  KtOutMax=[]  IntegratorOutMin=[]  IntegratorOutMax=[]  FilterOutMin=[]  FilterOutMax=[]  SumI1OutMin=[]  SumI1OutMax=[]  SumI2OutMin=[]  SumI2OutMax=[]  SumI3OutMin=[]  SumI3OutMax=[]  SumI4OutMin=[]  SumI4OutMax=[]  SumDOutMin=[]  SumDOutMax=[]  DifferentiatorOutMin=[]  DifferentiatorOutMax=[]  FilterDiffOutCoefMin=[]  FilterDiffOutCoefMax=[]  ReciprocalOutMin=[]  ReciprocalOutMax=[]  SumDenOutMin=[]  SumDenOutMax=[]  SumNumOutMin=[]  SumNumOutMax=[]  DivideOutMin=[]  DivideOutMax=[]  UdiffTsProdOutMin=[]  UdiffTsProdOutMax=[]  NTsProdOutMin=[]  NTsProdOutMax=[]  UintegralTsProdOutMin=[]  UintegralTsProdOutMax=[]  UngainTsProdOutMin=[]  UngainTsProdOutMax=[]  IntegratorContinuousStateAttributes='F_st'  IntegratorStateMustResolveToSignalObject=off  IntegratorRTWStateStorageClass=Auto  FilterContinuousStateAttributes=''  FilterStateMustResolveToSignalObject=off  FilterRTWStateStorageClass=Auto  ParallelPVariant=InternalParameters  IdealPVariant=Disabled  IVariant=InternalParameters  DVariant=Disabled  IntegratorVariant=Continuous  SatVariant=Disabled  AWVariant=Passthrough  PCopyVariant=Disabled  TRVariant=Disabled  FdbkBlocksVariant=Forward  IdealPFdbkVariant=Disabled  SatFdbkVariant=Disabled  DerivativeFilterVariant=Disabled  NVariant=Disabled  NCopyVariant=Disabled_SignalSpec  FilterICVariant=Disabled  IntegratorICVariant=InternalICs  ExternalResetVariant=Disabled  TRSumVariant=Passthrough  SumFdbkVariant=Disabled  SumVariant=Sum_PI  TsampFilterVariant=InternalTs  TsampNgainVariant=Passthrough  TsampIntegralVariant=Passthrough
  PID Controller5 : simulink/Continuous/PID Controller  Controller=PI  Form=Parallel  TimeDomain=Continuous-time  UseExternalTs=off  SampleTime=1  IntegratorMethod=Forward Euler  FilterMethod=Forward Euler  ControllerParametersSource=internal  P=cont_reg.Kp_AB_HHV  I=cont_reg.Ki_AB_HHV  D=0  UseFilter=on  N=100  TunerSelectOption=Transfer Function Based (PID Tuner App)  InitialConditionSource=internal  InitialConditionForIntegrator=0  InitialConditionForFilter=0  DifferentiatorICPrevScaledInput=0  ExternalReset=none  TrackingMode=off  Kt=1  LimitOutput=off  UpperSaturationLimit=inf  LowerSaturationLimit=-inf  LinearizeAsGain=on  AntiWindupMode=none  Kb=1  POutMin=[]  POutMax=[]  IOutMin=[]  IOutMax=[]  DOutMin=[]  DOutMax=[]  NOutMin=[]  NOutMax=[]  SumOutMin=[]  SumOutMax=[]  SaturationOutMin=[]  SaturationOutMax=[]  PParamMin=[]  PParamMax=[]  IParamMin=[]  IParamMax=[]  DParamMin=[]  DParamMax=[]  NParamMin=[]  NParamMax=[]  KbParamMin=[]  KbParamMax=[]  KtParamMin=[]  KtParamMax=[]  KbOutMin=[]  KbOutMax=[]  KtOutMin=[]  KtOutMax=[]  IntegratorOutMin=[]  IntegratorOutMax=[]  FilterOutMin=[]  FilterOutMax=[]  SumI1OutMin=[]  SumI1OutMax=[]  SumI2OutMin=[]  SumI2OutMax=[]  SumI3OutMin=[]  SumI3OutMax=[]  SumI4OutMin=[]  SumI4OutMax=[]  SumDOutMin=[]  SumDOutMax=[]  DifferentiatorOutMin=[]  DifferentiatorOutMax=[]  FilterDiffOutCoefMin=[]  FilterDiffOutCoefMax=[]  ReciprocalOutMin=[]  ReciprocalOutMax=[]  SumDenOutMin=[]  SumDenOutMax=[]  SumNumOutMin=[]  SumNumOutMax=[]  DivideOutMin=[]  DivideOutMax=[]  UdiffTsProdOutMin=[]  UdiffTsProdOutMax=[]  NTsProdOutMin=[]  NTsProdOutMax=[]  UintegralTsProdOutMin=[]  UintegralTsProdOutMax=[]  UngainTsProdOutMin=[]  UngainTsProdOutMax=[]  IntegratorContinuousStateAttributes=''  IntegratorStateMustResolveToSignalObject=off  IntegratorRTWStateStorageClass=Auto  FilterContinuousStateAttributes=''  FilterStateMustResolveToSignalObject=off  FilterRTWStateStorageClass=Auto  ParallelPVariant=InternalParameters  IdealPVariant=Disabled  IVariant=InternalParameters  DVariant=Disabled  IntegratorVariant=Continuous  SatVariant=Disabled  AWVariant=Passthrough  PCopyVariant=Disabled  TRVariant=Disabled  FdbkBlocksVariant=Forward  IdealPFdbkVariant=Disabled  SatFdbkVariant=Disabled  DerivativeFilterVariant=Disabled  NVariant=Disabled  NCopyVariant=Disabled_SignalSpec  FilterICVariant=Disabled  IntegratorICVariant=InternalICs  ExternalResetVariant=Disabled  TRSumVariant=Passthrough  SumFdbkVariant=Disabled  SumVariant=Sum_PI  TsampFilterVariant=InternalTs  TsampNgainVariant=Passthrough  TsampIntegralVariant=Passthrough
  Scope : Scope
  Scope1 : Scope
  Scope2 : Scope
  Sum{,2..4} (4 alike) : Sum  Inputs=+-|
  Sum1 : Sum  Commented=on  Inputs=-+|
  Sum{10..11,14..15} (4 alike) : Sum  Inputs=++|
  Sum{9,12..13,16} (4 alike) : Sum  Inputs=|++
  Sum{8,17..19} (4 alike) : Sum  Commented=on  Inputs=++|
  Sum5 : Sum  Commented=on  Inputs=|+-
  Sum6 : Sum  Commented=on  Inputs=-+|
  Sum7 : Sum  Commented=on  Inputs=|+-
  Unit Delay : UnitDelay  Commented=on  HasFrameUpgradeWarning=on
  Unit Delay1 : UnitDelay  Commented=on  HasFrameUpgradeWarning=on
  st_PID_LPF : TransferFcn  Denominator=[cont_reg.T_st_LPF^2 sqrt(2)*cont_reg.T_st_LPF 1]
  st_PID_LPF1 : TransferFcn  Denominator=[cont_reg.T_AB_LPF^2 sqrt(2)*cont_reg.T_AB_LPF 1]
  st_PID_LPF2 : TransferFcn  Denominator=[cont_reg.T_st_LPF^2 sqrt(2)*cont_reg.T_st_LPF 1]
  st_PID_LPF3 : TransferFcn  Denominator=[cont_reg.T_AB_LPF^2 sqrt(2)*cont_reg.T_AB_LPF 1]
  st_PID_LPF{4..7} (4 alike) : TransferFcn  Commented=on  Denominator=[reg.T_MPC_LPF 1]
  F_aII_out : Outport  VectorParamsAs1DForOutWhenUnconnected=off
  Fi_aI_out : Outport  Port=2  VectorParamsAs1DForOutWhenUnconnected=off
  v_grate_out : Outport  Port=3  VectorParamsAs1DForOutWhenUnconnected=off
  Fi_w_out : Outport  Port=4  VectorParamsAs1DForOutWhenUnconnected=off
  wires:
  Multiply4/1 -> Sum15/2
  Multiply3/1 -> Sum11/2
  Sum19/1 -> Controller selector 3/3(mpc)
  Sum18/1 -> Controller selector 2/3(mpc)
  Sum8/1 -> "Controller selector "/3(mpc)
  Sum17/1 -> Controller selector 1/3(mpc)
  Constant36/1 -> Sum19/1
  Constant35/1 -> Sum18/1
  Constant15/1 -> Sum17/1
  Constant34/1 -> Sum8/1
  st_PID_LPF7/1 -> Sum19/2
  st_PID_LPF6/1 -> Sum18/2
  st_PID_LPF5/1 -> Sum17/2
  st_PID_LPF4/1 -> Sum8/2
  Unit Delay1/1 -> Sum7/1
  Unit Delay/1 -> Sum6/2
  Sum16/1 -> Controller selector 3/2(cascade)  "F_aI_CPID"
  Sum15/1 -> Controller selector 2/2(cascade)
  Multiply1/1 -> Sum16/1
  Constant32/1 -> Sum15/1
  Constant33/1 -> Sum16/2
  PID Controller5/1 -> st_PID_LPF3/1
  st_PID_LPF3/1 -> Multiply1/1, Multiply4/1
  Constant30/1 -> Controller selector 3/4(controller_type)
  Constant13/1 -> Controller selector 2/4(controller_type)
  Constant29/1 -> Controller selector 1/4(controller_type)
  Constant31/1 -> "Controller selector "/4(controller_type)
  Constant1/1 -> Sum14/1
  O2_PID_LPF/1 -> Sum14/2
  Constant9/1 -> Sum13/2
  Constant28/1 -> Sum9/2
  Sum6/1 -> Mux/1
  Sum1/1 -> Mux1/1
  st_PID_LPF2/1 -> Sum9/1
  Sum10/1 -> Sum/1
  Constant21/1 -> Sum10/1
  Multiply/1 -> Sum10/2
  PID Controller2/1 -> Multiply/1, Scope2/1  "sp_HHV"
  Sum9/1 -> Controller selector 1/2(cascade)
  PID Controller1/1 -> st_PID_LPF2/1  "ABC_F_aI_out"
  Sum12/1 -> Controller selector 3/1(ab)  "F_aI_CPID"
  Constant27/1 -> Input  selector4/1(constant), Input  selector4/2(experimental)
  Input  selector1/1(signal) -> PID Controller2/1, PID Controller3/1  "F_st"
  Constant26/1 -> Input  selector1/1(constant), Input  selector1/2(experimental)
  Constant6/1 -> Input  selector1/4(input_type)
  Sum3/1 -> Input  selector1/3(controlled)
  Constant25/1 -> Input  selector/1(constant), Input  selector/2(experimental)
  Sum2/1 -> Input  selector/3(controlled)
  Constant24/1 -> Input  selector2/1(constant), Input  selector2/2(experimental)
  Input  selector2/1(signal) -> PID Controller/1, PID Controller5/1
  Sum4/1 -> Input  selector2/3(controlled)
  Divide/1 -> Sum4/2  "A/B"
  Constant23/1 -> Input  selector5/1(constant), Input  selector5/2(experimental)
  Sum/1 -> Input  selector5/3(controlled)  "ABC_e_HHV"
  Constant22/1 -> Input  selector5/4(input_type)
  Input  selector5/1(signal) -> PID Controller1/1  "ABC_e_HHV"
  HHV_in/1 -> Sum/2  "HHV_in"
  Constant20/1 -> Input  selector3/1(constant), Input  selector3/2(experimental)
  Input  selector4/1(signal) -> MPC/2
  Mux1/1 -> Input  selector4/3(controlled)
  Constant19/1 -> Input  selector4/4(input_type)
  Constant18/1 -> Input  selector3/4(input_type)
  Mux/1 -> Input  selector3/3(controlled)
  Input  selector3/1(signal) -> MPC/1
  Constant17/1 -> Sum7/2
  Constant16/1 -> Sum6/1
  Sum7/1 -> Mux/2
  MPC/1 -> Demux/1
  Sum5/1 -> Mux1/2
  Constant14/1 -> Sum5/2
  Constant11/1 -> Sum5/1
  Constant/1 -> Sum1/1
  Constant12/1 -> Sum1/2
  Controller selector 3/1(signal) -> Fi_w_out/1  "F_w_in"
  Controller selector 2/1(signal) -> v_grate_out/1  "v_grate"
  Controller selector 1/1(signal) -> Fi_aI_out/1, Divide/1  "F_aI"
  "Controller selector "/1(signal) -> F_aII_out/1, Divide/2  "F_aII"
  Demux/4 -> st_PID_LPF7/1
  Demux/3 -> st_PID_LPF6/1
  Demux/2 -> st_PID_LPF5/1
  Demux/1 -> st_PID_LPF4/1
  st_PID_LPF1/1 -> Multiply3/1, Multiply2/1
  st_PID_LPF/1 -> Sum13/1
  Constant10/1 -> Sum11/1
  Multiply2/1 -> Sum12/1
  Sum11/1 -> Controller selector 2/1(ab)
  PID Controller/1 -> st_PID_LPF1/1
  Constant8/1 -> Sum12/2
  Sum13/1 -> Controller selector 1/1(ab)
  PID Controller3/1 -> st_PID_LPF/1, Scope1/1
  Sum14/1 -> "Controller selector "/2(cascade), "Controller selector "/1(ab)
  PID Controller4/1 -> O2_PID_LPF/1, Scope/1
  "F_O2_in (Expected 14 values, new simulator does not use that (?))"/1 -> Sum2/2, Unit Delay/1  "F_O2_in"
  Constant3/1 -> Sum3/1
  F_st_in/1 -> Sum3/2, Unit Delay1/1  "F_st_in"
  Constant2/1 -> Sum2/1
  Fi_fg_in/1 -> "F_O2_in (Expected 14 values, new simulator does not use that (?))"/1  "Fi_fg_in"
  Constant4/1 -> Sum4/1
  Constant5/1 -> Input  selector/4(input_type)
  Constant7/1 -> Input  selector2/4(input_type)
  Input  selector/1(signal) -> PID Controller4/1  "F_O2"

== system Furnace/Deprecated, slow loop/Contineous Summer student feedback (Not finished)/Grate speed ==
  v_grate_reg_in : Inport
  Constant : Constant  Commented=on  Value=cont_reg.const_Q_grate
  Constant1 : Constant  Value=cont_reg.input_type_v_grate
  Constant2 : Constant  Commented=on  Value=cont_reg.input_type_Q_grate
  From Workspace2 : FromWorkspace  Commented=on  VariableName=Q_grate
  Input selector1 : MATLAB Function  TreatAsAtomicUnit=on
  Input selector2 : MATLAB Function  Commented=on  TreatAsAtomicUnit=on
  const_Q_grate : Constant  Commented=on  Value=cont_reg.const_Q_grate
  const_v_grate : Constant  Value=cont_reg.const_v_grate
  v_grate : Constant  Value=k.v_grate
  v_grate_out : Outport  VectorParamsAs1DForOutWhenUnconnected=off
  Q_grate_out : Outport  Port=2  VectorParamsAs1DForOutWhenUnconnected=off
  wires:
  Constant/1 -> Input selector2/3(controlled)
  From Workspace2/1 -> Input selector2/2(experimental)
  Constant2/1 -> Input selector2/4(input_type)
  const_Q_grate/1 -> Input selector2/1(constant)  "const_Q_grate"
  const_v_grate/1 -> Input selector1/1(constant)  "const_v_grate"
  v_grate_reg_in/1 -> Input selector1/3(controlled)
  Constant1/1 -> Input selector1/4(input_type)
  Input selector1/1(signal) -> v_grate_out/1  "v_grate"
  v_grate/1 -> Input selector1/2(experimental)
  Input selector2/1(signal) -> Q_grate_out/1  "Q_grate"

== system Furnace/Deprecated, slow loop/Contineous Summer student feedback (Not finished)/Secondary air ==
  F_aII_reg_in : Inport
  Constant : Constant  Value=cont_reg.input_type_F_aII
  Constant2 : Constant  Commented=on  Value=reg.const_T_aII
  Constant3 : Constant  Commented=on  Value=reg.input_type_T_aII
  Flue gas fan : Subsystem
  From Workspace1 : FromWorkspace  Commented=on  VariableName=F_aII
  Goto : Goto  Commented=on  GotoTag=F_aII  TagVisibility=global
  Goto1 : Goto  Commented=on  GotoTag=T_aII  TagVisibility=global
  Input  selector : MATLAB Function  TreatAsAtomicUnit=on
  Input  selector1 : MATLAB Function  Commented=on  TreatAsAtomicUnit=on
  PID Controller : simulink/Continuous/PID Controller  Controller=PI  Form=Parallel  TimeDomain=Continuous-time  UseExternalTs=off  SampleTime=1  IntegratorMethod=Forward Euler  FilterMethod=Forward Euler  ControllerParametersSource=internal  P=cont_reg.Kp_fan  I=cont_reg.Ki_fan  D=0  UseFilter=on  N=100  TunerSelectOption=Transfer Function Based (PID Tuner App)  InitialConditionSource=internal  InitialConditionForIntegrator=cont_reg.F_aII_fan_PID_int  InitialConditionForFilter=0  DifferentiatorICPrevScaledInput=0  ExternalReset=none  TrackingMode=off  Kt=1  LimitOutput=off  UpperSaturationLimit=inf  LowerSaturationLimit=-inf  LinearizeAsGain=on  AntiWindupMode=none  Kb=1  POutMin=[]  POutMax=[]  IOutMin=[]  IOutMax=[]  DOutMin=[]  DOutMax=[]  NOutMin=[]  NOutMax=[]  SumOutMin=[]  SumOutMax=[]  SaturationOutMin=[]  SaturationOutMax=[]  PParamMin=[]  PParamMax=[]  IParamMin=[]  IParamMax=[]  DParamMin=[]  DParamMax=[]  NParamMin=[]  NParamMax=[]  KbParamMin=[]  KbParamMax=[]  KtParamMin=[]  KtParamMax=[]  KbOutMin=[]  KbOutMax=[]  KtOutMin=[]  KtOutMax=[]  IntegratorOutMin=[]  IntegratorOutMax=[]  FilterOutMin=[]  FilterOutMax=[]  SumI1OutMin=[]  SumI1OutMax=[]  SumI2OutMin=[]  SumI2OutMax=[]  SumI3OutMin=[]  SumI3OutMax=[]  SumI4OutMin=[]  SumI4OutMax=[]  SumDOutMin=[]  SumDOutMax=[]  DifferentiatorOutMin=[]  DifferentiatorOutMax=[]  FilterDiffOutCoefMin=[]  FilterDiffOutCoefMax=[]  ReciprocalOutMin=[]  ReciprocalOutMax=[]  SumDenOutMin=[]  SumDenOutMax=[]  SumNumOutMin=[]  SumNumOutMax=[]  DivideOutMin=[]  DivideOutMax=[]  UdiffTsProdOutMin=[]  UdiffTsProdOutMax=[]  NTsProdOutMin=[]  NTsProdOutMax=[]  UintegralTsProdOutMin=[]  UintegralTsProdOutMax=[]  UngainTsProdOutMin=[]  UngainTsProdOutMax=[]  IntegratorContinuousStateAttributes=''  IntegratorStateMustResolveToSignalObject=off  IntegratorRTWStateStorageClass=Auto  FilterContinuousStateAttributes=''  FilterStateMustResolveToSignalObject=off  FilterRTWStateStorageClass=Auto  ParallelPVariant=InternalParameters  IdealPVariant=Disabled  IVariant=InternalParameters  DVariant=Disabled  IntegratorVariant=Continuous  SatVariant=Disabled  AWVariant=Passthrough  PCopyVariant=Disabled  TRVariant=Disabled  FdbkBlocksVariant=Forward  IdealPFdbkVariant=Disabled  SatFdbkVariant=Disabled  DerivativeFilterVariant=Disabled  NVariant=Disabled  NCopyVariant=Disabled_SignalSpec  FilterICVariant=Disabled  IntegratorICVariant=InternalICs  ExternalResetVariant=Disabled  TRSumVariant=Passthrough  SumFdbkVariant=Disabled  SumVariant=Sum_PI  TsampFilterVariant=InternalTs  TsampNgainVariant=Passthrough  TsampIntegralVariant=Passthrough
  Sum1 : Sum  Inputs=|+-
  T_aII : FromWorkspace  Commented=on  VariableName=T_aII
  Terminator : Terminator
  Terminator1 : Terminator
  const_F_aII : Constant  Value=cont_reg.const_F_aII
  F_aII_out : Outport  VectorParamsAs1DForOutWhenUnconnected=off
  F_aII_out1 : Outport  Port=2  VectorParamsAs1DForOutWhenUnconnected=off
  wires:
  Flue gas fan/3(Power consumption) -> Terminator1/1
  Flue gas fan/2(Pressure difference) -> Terminator/1
  Flue gas fan/1(Volume flow) -> Sum1/2, F_aII_out/1, Goto/1
  Input  selector/1(signal) -> Sum1/1  "F_aII"
  PID Controller/1 -> Flue gas fan/1(PID signal)
  Sum1/1 -> PID Controller/1
  Input  selector1/1(signal) -> F_aII_out1/1, Goto1/1
  Constant3/1 -> Input  selector1/4(input_type)
  Constant/1 -> Input  selector/4(input_type)
  const_F_aII/1 -> Input  selector/1(constant)  "const_F_aII"
  From Workspace1/1 -> Input  selector/2(experimental)
  F_aII_reg_in/1 -> Input  selector/3(controlled)
  T_aII/1 -> Input  selector1/2(experimental)
  Constant2/1 -> Input  selector1/1(constant)
